simulink model "sl_ctorqueTraj"  (R2014a)
settings: Solver=ode45  StartTime=0.0  StopTime=10  FixedStep=0.01  MaxStep=0.05  RelTol=1e-3
PreLoadFcn:
  | puma560
  | p560 = nofriction(p560);
libraries: roblocks x7
settings Model: ExtModeTrigMode=oneshot  ExtModeArmWhenConnect=off  Creator=pic  LastModifiedBy=MRDLAB
settings SolverCC: ZeroCrossControl=DisableAll
settings DataIOCC: LimitDataPoints=off  SignalLoggingSaveFormat=ModelDataLogs  ReturnWorkspaceOutputs=on
settings OptimizationCC: BlockReduction=off  BooleanDataType=off  ExpressionDepthLimit=2147483647  InitFltsAndDblsToZero=on
settings DebuggingCC: SaveWithParameterizedLinksMsg=none  UnderspecifiedInitializationDetection=Classic  SignalResolutionControl=TryResolveAllWithWarning  SolverPrmCheckMsg=none  MultiTaskDSMMsg=warning  MultiTaskCondExecSysMsg=none  FcnCallInpInsideContextMsg=UseLocalSettings  StateNameClashWarn=warning
settings HardwareCC: TargetUnknown=on
settings RTWCC: IncludeERTFirstTime=on
settings GRTTargetCC: ModelReferenceCompliant=off  CompOptLevelCompliant=off  CombineOutputUpdateFcns=off  MatFileLogging=off  GRTInterface=on

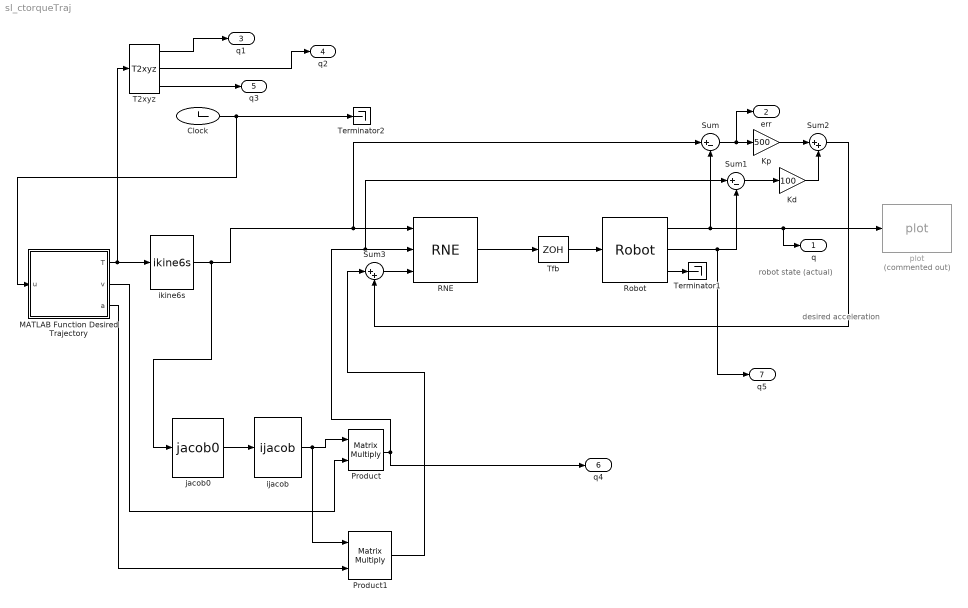
== system sl_ctorqueTraj ==
  note: robot state
      | (actual)
  note: desired acceleration
  Clock : Clock
  Kd : Gain  Gain=100  SaturateOnIntegerOverflow=on  OutDataTypeStr=Inherit: Same as input  ParamDataTypeStr=Inherit: Same as input
  Kp : Gain  Gain=500  SaturateOnIntegerOverflow=on  OutDataTypeStr=Inherit: Same as input  ParamDataTypeStr=Inherit: Same as input
  MATLAB Function Desired Trajectory : MATLAB Function  TreatAsAtomicUnit=on
  Product : Product  Multiplication=Matrix(*)
  Product1 : Product  Multiplication=Matrix(*)
  RNE : roblocks/Dynamics/RNE  robot=myRobot  grav=[0 0 9.81]
  Robot : roblocks/Dynamics/Robot  robot=myRobot  q0="[2.9083    1.6809   -0.1451     -0.9350   -0.9404   -2.9065]"
  Sum : Sum  Inputs=|+-  SaturateOnIntegerOverflow=on  InputSameDT=on  OutDataTypeStr=Inherit: Same as first input
  Sum1 : Sum  Inputs=|+-  SaturateOnIntegerOverflow=on  InputSameDT=on  OutDataTypeStr=Inherit: Same as first input
  Sum2 : Sum  Inputs=|++  SaturateOnIntegerOverflow=on  InputSameDT=on  OutDataTypeStr=Inherit: Same as first input
  Sum3 : Sum  Inputs=|++  SaturateOnIntegerOverflow=on  InputSameDT=on  OutDataTypeStr=Inherit: Same as first input
  T2xyz : roblocks/Transform Conversion/T2xyz
  Terminator1 : Terminator
  Terminator2 : Terminator
  Tfb : ZeroOrderHold  SampleTime=0.01
  ijacob : roblocks/Kinematics/ijacob
  ikine6s : roblocks/Kinematics/ikine6s  robot=myRobot  conf='luf'
  "jacob0 " : roblocks/Kinematics/jacob0   robot=myRobot
  plot : roblocks/Robot Graphics/plot  Commented=on  robot=myRobot  fps=25  holdplot=on
  q : Outport
  err : Outport  Port=2
  q1 : Outport  Port=3
  q2 : Outport  Port=4
  q3 : Outport  Port=5
  q4 : Outport  Port=6
  q5 : Outport  Port=7
  wires:
  Sum/1 -> Kp/1, err/1
  Kp/1 -> Sum2/1
  Robot/1 -> Sum/2, q/1, plot/1
  Robot/2 -> q5/1, Sum1/2
  RNE/1 -> Tfb/1
  ikine6s/1 -> "jacob0 "/1, Sum/1, RNE/1
  Product/1 -> RNE/2, Sum1/1, q4/1
  Sum1/1 -> Kd/1
  Kd/1 -> Sum2/2
  Product1/1 -> Sum3/1
  Robot/3 -> Terminator1/1
  Clock/1 -> MATLAB Function Desired Trajectory/1(u), Terminator2/1
  Sum3/1 -> RNE/3
  Sum2/1 -> Sum3/2
  Tfb/1 -> Robot/1
  MATLAB Function Desired Trajectory/1(T) -> T2xyz/1, ikine6s/1
  "jacob0 "/1 -> ijacob/1
  ijacob/1 -> Product1/1, Product/1
  MATLAB Function Desired Trajectory/2(v) -> Product/2
  MATLAB Function Desired Trajectory/3(a) -> Product1/2
  T2xyz/1 -> q1/1
  T2xyz/3 -> q3/1
  T2xyz/2 -> q2/1

== matlab function sl_ctorqueTraj/MATLAB Function Desired Trajectory ==
  data: u input; T output; v output; a output
% writen by Rod Dockter
% Allows creation of a trajectory as a function of time out put to a
% transformation matrix
% Fixes the problems in tims code
function [T,v,a]  = desiredTrajectory(u)

 
 
t = u(1);         % sample time
A = 0.05;         % circle radius in meters
k = 2*pi;         % angular freq. < ---- This changes your speed.
x0= .5;
z0= .5;

MoveAlong=[ 0.7071         0    0.7071    0.5000;
           -0.5000    0.7071    0.5000         0;
           -0.5000   -0.7071    0.5000    0.5000;
                 0         0         0    1.0000];
JustRot  =[    0.7071         0    0.7071         0;
               -0.5000    0.7071    0.5000         0;
               -0.5000   -0.7071    0.5000         0;
                     0         0         0    1.0000];

T= [1 0 0 A*sin(k*t);
    0 1 0 A*cos(k*t);
    0 0 1 0;
    0 0 0 1];
T=MoveAlong*T;


vtemp=[    k*A*cos(k*t)    -k*A*sin(k*t)   0 0]';
vtemp=JustRot*vtemp;
v=[vtemp;0;0];


atemp=[ -k^2*A*sin(k*t)  -k^2*A*cos(k*t)   0 0]';
atemp=JustRot*atemp;
a=[atemp;0;0];


%               x                y        z  | orientation
%q = myRobot.ikine(6)
%q   = [      A*sin(k*t)       A*cos(k*t)  z0     0 0 0   ]'; 
%qd  = [    k*A*cos(k*t)    -k*A*sin(k*t)   0     0 0 0   ]'; 
%qdd = [ -k^2*A*sin(k*t)  -k^2*A*cos(k*t)   0     0 0 0   ]';
